simulink model "Motor_Model_NoControl"  (R2024b)
settings: Solver=VariableStepAuto  StartTime=0.0  StopTime=0.37  RelTol=1e-3
libraries: fl_lib x16, nesl_utility x7, ee_lib x2
settings Model: Creator=rubse  LastModifiedBy=Mischa Johal
settings SolverCC: AlgebraicLoopSolver=TrustRegion
settings DebuggingCC: UnconnectedInputMsg=warning  UnconnectedOutputMsg=warning  UnconnectedLineMsg=warning
settings ModelReferenceCC: EnableRefExpFcnMdlSchedulingChecks=on
settings RTWCC: GPUComputeCapability=3.5  DLArmComputeVersion=19.05

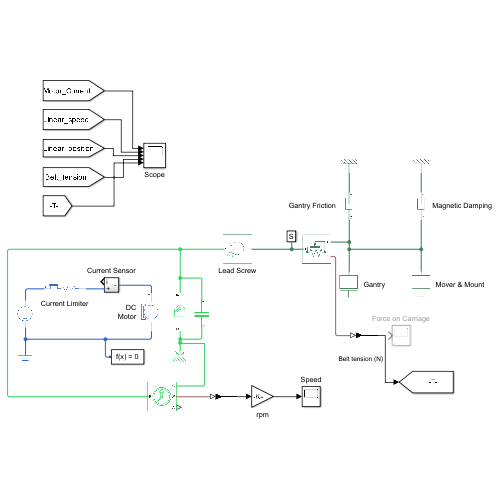
[thumbnail: Simulink's stored preview of the top-level diagram]
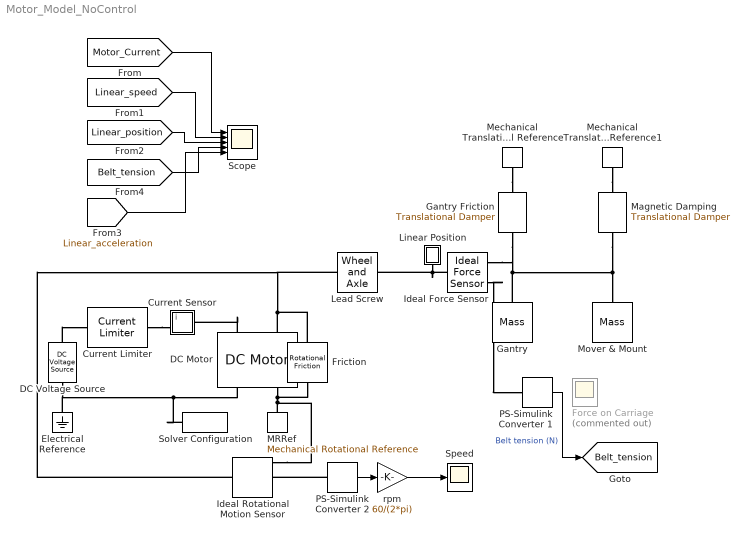
== system Motor_Model_NoControl ==
  Current Limiter : ee_lib/Semiconductors & Converters/Current Limiter  limType=ee.enum.semiconductors.currLimType.constLim  iLim=40 A  iLimReverse=1 A  vLim=0.1 V  gLim=1e-3 1/Ohm  thermal_mass=100 J/K  temperature_specify=off  temperature_priority=High  temperature=298.15 K  temperature_nominal_specify=off  temperature_nominal_value=1  temperature_nominal_unit=K
      settings: InternalSimscapePortConfiguration="{\"Bottom\":[],\"Left\":[{\"id\":\"p\",\"label\":\"+\",\"type\":\"foundation.electrical.electrical\"}],\"Right\":[{\"id\":\"n\",\"label\":\"-\",\"type\":\"foundation.electrical.electrical\"}],\"Top\":[]}"
  Current Sensor : Subsystem
  DC Motor : ee_lib/Electromechanical/Brushed Motors/DC Motor  field_option=ee.enum.field_option.pm  Rf=100 Ohm  Lf=1 H  Laf=0.15 H  If0=0 A  parameterization=ee.enum.dcparam_option.load_speed  Ra=0.0787 Ohm  La=12e-6 H  emf_or_torque=ee.enum.emf_or_torque.ki  Kv=0.0637 V/rpm  Ki=32.3e-3 N*m/A  T_stall=2.4e-4 N*m  w_max=3500 rpm  w_rated=2970 rpm  P_rated=350 W  V_rated=24 V  lam_param=ee.enum.lam_param.current  i_noload=1.3 A  V_i_noload=24 V  J=3530.77 g*cm^2  lam=1e-08 N*m/(rad/s)  speed0=392 rpm  t_fault_armature=1 s  t_fault_field=1 s  fault_action=simscape.enum.assert.action.none  alpha=3.93e-3 1/K  Tmeas=25 degC  thermal_mass=100 J/K  initial_temperature=25 degC
  DC Voltage Source : fl_lib/Electrical/Electrical Sources/DC Voltage Source  v0=0 V
  Electrical Reference : fl_lib/Electrical/Electrical Elements/Electrical Reference
  Force on Carriage : Scope  Commented=on
  Friction : fl_lib/Mechanical/Rotational Elements/Rotational Friction  brkwy_trq=0.06565 N*m  brkwy_vel=0.03347 rad/s  Col_trq=0.022 N*m  visc_coef=0 N*m/(rad/s)  w_specify=off  w_priority=High  w=0 rad/s  w_nominal_specify=off  w_nominal_value=1  w_nominal_unit=rad/s  t_specify=off  t_priority=High  t=0 N*m  t_nominal_specify=off  t_nominal_value=1  t_nominal_unit=N*m
  Gantry : fl_lib/Mechanical/Translational Elements/Mass  mass=4.5 kg  num_ports=foundation.enum.numPorts2.one  v_specify=off  v_priority=High  v=0 m/s  v_nominal_specify=off  v_nominal_value=1  v_nominal_unit=m/s  f_specify=off  f_priority=None  f=0 N  f_nominal_specify=off  f_nominal_value=1  f_nominal_unit=N
  Gantry Friction : fl_lib/Mechanical/Translational Elements/Translational Damper  D=0.09 N/(m/s)  v_specify=off  v_priority=None  v=0 m/s  v_nominal_specify=off  v_nominal_value=1  v_nominal_unit=m/s  f_specify=off  f_priority=None  f=0 N  f_nominal_specify=off  f_nominal_value=1  f_nominal_unit=N
  Ideal Force Sensor : fl_lib/Mechanical/Mechanical Sensors/Ideal Force Sensor
  Ideal Rotational Motion Sensor : fl_lib/Mechanical/Mechanical Sensors/Ideal Rotational Motion Sensor  reference=foundation.enum.MeasurementReference.difference  acceleration_port=false  velocity_port=true  position_port=true  wrap_angle=simscape.enum.onoff.off  offset=0 rad
  Lead Screw : fl_lib/Mechanical/Mechanisms/Wheel and Axle  R=0.05 m  or=1  t_specify=off  t_priority=High  t=0 N*m  t_nominal_specify=off  t_nominal_value=1  t_nominal_unit=N*m  f_specify=off  f_priority=High  f=0 N  f_nominal_specify=off  f_nominal_value=1  f_nominal_unit=N
  Linear Position : Subsystem
      mask Display: disp('S');
  MRRef : fl_lib/Mechanical/Rotational Elements/Mechanical Rotational Reference
  Magnetic Damping : fl_lib/Mechanical/Translational Elements/Translational Damper  D=5 N/(m/s)  v_specify=off  v_priority=None  v=0 m/s  v_nominal_specify=off  v_nominal_value=1  v_nominal_unit=m/s  f_specify=off  f_priority=None  f=0 N  f_nominal_specify=off  f_nominal_value=1  f_nominal_unit=N
  Mechanical Translational Reference : fl_lib/Mechanical/Translational Elements/Mechanical Translational Reference
  Mechanical Translational Reference1 : fl_lib/Mechanical/Translational Elements/Mechanical Translational Reference
  Mover & Mount : fl_lib/Mechanical/Translational Elements/Mass  mass=1.5 kg  num_ports=foundation.enum.numPorts2.one  v_specify=off  v_priority=High  v=0 m/s  v_nominal_specify=off  v_nominal_value=1  v_nominal_unit=m/s  f_specify=off  f_priority=None  f=0 N  f_nominal_specify=off  f_nominal_value=1  f_nominal_unit=N
  PS-Simulink Converter 1 : nesl_utility/PS-Simulink Converter  PhysicalDomain=network_engine_domain  SubClassName=ps_output  LeftPortType=input  RightPortType=output  PseudoPeriodic=off  Frequencies=[]  VectorFormat=1-D array  Unit=N  AffineConversion=off
  PS-Simulink Converter 2 : nesl_utility/PS-Simulink Converter  PhysicalDomain=network_engine_domain  SubClassName=ps_output  LeftPortType=input  RightPortType=output  PseudoPeriodic=off  Frequencies=[]  VectorFormat=1-D array  Unit=rad/s  AffineConversion=off
  Scope : Scope  NumInputPorts=5
  Solver Configuration : nesl_utility/Solver Configuration  PhysicalDomain=network_engine_domain  SubClassName=solver  LeftPortType=input  RightPortType=generic  Tones=[]  Harmonics=[]  SimulateNoise=off  Profile=off  UseLocalSampling=off  EnableSwitchedLinearOptims=on  FrequencyDomain=off  UseCCode=off  RelTol=0.001  AbsTol=1e-06  MinStep=1e-09  ToWorkspace=off  RevertToSquareIcSolve=off  NumHomotopyIterations=100  PhasorMode=off  PhasorModeNumHarmonics=1  ConsistencySolver=NEWTON_FTOL  IndexReductionMethod=DerivativeReplacement  DoDC=off  ResidualTolerance=1e-9  ConsistencyTolSource=GLOBAL  ConsistencyAbsTol=0.001  ConsistencyRelTol=0.001  ConsistencyTolFactor=0.001  UseLocalSolver=off  LocalSolverChoice=NE_BACKWARD_EULER_ADVANCER  ResolveIndetEquations=on  FunctionEvalNumThread=1  LocalSolverSampleTime=0.0001  DoFixedCost=off  MaxNonlinIter=3  MaxModeIter=2  ComputeImpulses=off  ImpulseIterations=2  LinearAlgebra=auto  LinearAlgebraNumThread=0  EquationFormulation=NE_TIME_EF  DelaysMemoryBudget=1024  AutomaticFiltering=on  FilteringTimeConstant=0.001  PartitionStorageMethod=AS_NEEDED  PartitionMemoryBudget=1024  PartitionMethod=FAST  MultibodyUseLocalSolver=off  MultibodyLocalSolverChoice=ODE1  MultibodyLocalSolverSampleTime=0.001
  Speed : Scope
  rpm : Gain  Gain=60/(2*pi)
  tag scope: Belt_tension=global
  wires:
  PS-Simulink Converter 2/1 -> rpm/1
  rpm/1 -> Speed/1
  PS-Simulink Converter 1/1 -> [Belt_tension]  "Belt tension (N)"
  [Motor_Current] -> Scope/1
  [Linear_speed] -> Scope/2
  [Linear_position] -> Scope/3
  [Belt_tension] -> Scope/4
  [Linear_acceleration] -> Scope/5
  connections:
  DC Motor/RConn2 -- MRRef/LConn1 -- Friction/RConn1 -- Ideal Rotational Motion Sensor/RConn1
  DC Motor/LConn2 -- Ideal Rotational Motion Sensor/LConn1 -- Lead Screw/LConn1 -- Friction/LConn1
  Linear Position/LConn1 -- Ideal Force Sensor/LConn1 -- Lead Screw/RConn1
  Solver Configuration/RConn1 -- Electrical Reference/LConn1 -- DC Voltage Source/RConn1 -- DC Motor/RConn1
  DC Motor/LConn1 -- Current Sensor/LConn1
  Mechanical Translational Reference/LConn1 -- Gantry Friction/LConn1
  Gantry/LConn1 -- Mover & Mount/LConn1 -- Magnetic Damping/RConn1 -- Ideal Force Sensor/RConn1 -- Gantry Friction/RConn1
  Mechanical Translational Reference1/LConn1 -- Magnetic Damping/LConn1
  PS-Simulink Converter 2/LConn1 -- Ideal Rotational Motion Sensor/RConn2
  Ideal Force Sensor/RConn2 -- PS-Simulink Converter 1/LConn1
  DC Voltage Source/LConn1 -- Current Limiter/LConn1
  Current Limiter/RConn1 -- Current Sensor/RConn1

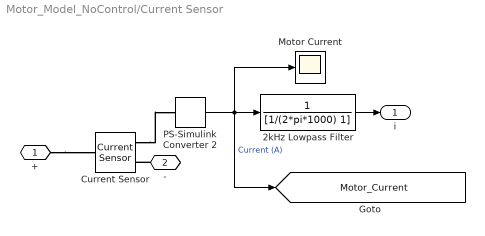
== system Motor_Model_NoControl/Current Sensor ==
  2kHz Lowpass Filter : TransferFcn  Denominator=[1/(2*pi*1000) 1]
  Current Sensor : fl_lib/Electrical/Electrical Sensors/Current Sensor
  Motor Current : Scope
  PS-Simulink Converter 2 : nesl_utility/PS-Simulink Converter  PhysicalDomain=network_engine_domain  SubClassName=ps_output  LeftPortType=input  RightPortType=output  PseudoPeriodic=off  Frequencies=[]  VectorFormat=1-D array  Unit=A  AffineConversion=off
  + : PMIOPort  Side=Right
  - : PMIOPort  Port=2  Side=Left
  i : Outport  VectorParamsAs1DForOutWhenUnconnected=off
  tag scope: Motor_Current=global
  wires:
  PS-Simulink Converter 2/1 -> [Motor_Current], 2kHz Lowpass Filter/1, Motor Current/1  "Current (A)"
  2kHz Lowpass Filter/1 -> i/1
  connections:
  +/RConn1 -- Current Sensor/LConn1
  -/RConn1 -- Current Sensor/RConn2
  Current Sensor/RConn1 -- PS-Simulink Converter 2/LConn1

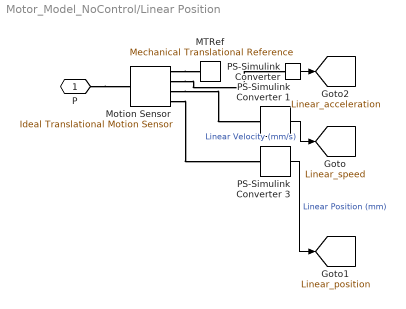
== system Motor_Model_NoControl/Linear Position ==
  MTRef : fl_lib/Mechanical/Translational Elements/Mechanical Translational Reference
  Motion Sensor : fl_lib/Mechanical/Mechanical Sensors/Ideal Translational Motion Sensor  reference=foundation.enum.MeasurementReference.difference  acceleration_port=true  velocity_port=true  position_port=true  offset=0 m
      settings: InternalSimscapePortConfiguration="{\"Bottom\":[],\"Left\":[{\"id\":\"R\",\"label\":\"R\",\"type\":\"foundation.mechanical.translational.translational\"}],\"Right\":[{\"id\":\"C\",\"label\":\"C\",\"type\":\"foundation.mechanical.translational.translational\"},{\"id\":\"A\",\"label\":\"A\",\"type\":\"output\"},{\"id\":\"V\",\"label\":\"V\",\"type\":\"output\"},{\"id\":\"P\",\"label\":\"P\",\"type\":\"output\"}],\"Top\":[]}"
  PS-Simulink Converter : nesl_utility/PS-Simulink Converter  PhysicalDomain=network_engine_domain  SubClassName=ps_output  LeftPortType=input  RightPortType=output  PseudoPeriodic=off  Frequencies=[]  VectorFormat=1-D array  Unit=mm/s^2  AffineConversion=off
  PS-Simulink Converter 1 : nesl_utility/PS-Simulink Converter  PhysicalDomain=network_engine_domain  SubClassName=ps_output  LeftPortType=input  RightPortType=output  PseudoPeriodic=off  Frequencies=[]  VectorFormat=1-D array  Unit=mm/s  AffineConversion=off
  PS-Simulink Converter 3 : nesl_utility/PS-Simulink Converter  PhysicalDomain=network_engine_domain  SubClassName=ps_output  LeftPortType=input  RightPortType=output  PseudoPeriodic=off  Frequencies=[]  VectorFormat=1-D array  Unit=mm  AffineConversion=off
  P : PMIOPort  Side=Left
  tag scope: Linear_acceleration=global, Linear_position=global, Linear_speed=global
  wires:
  PS-Simulink Converter 3/1 -> [Linear_position]  "Linear Position (mm)"
  PS-Simulink Converter 1/1 -> [Linear_speed]  "Linear Velocity (mm/s)"
  PS-Simulink Converter/1 -> [Linear_acceleration]
  connections:
  Motion Sensor/RConn1 -- MTRef/LConn1
  Motion Sensor/RConn4 -- PS-Simulink Converter 3/LConn1
  P/RConn1 -- Motion Sensor/LConn1
  Motion Sensor/RConn3 -- PS-Simulink Converter 1/LConn1
  Motion Sensor/RConn2 -- PS-Simulink Converter/LConn1
